simulink model "test_dca"  (R2018a)
settings: Solver=FixedStepAuto  StartTime=0.0  StopTime=4  FixedStep=0.01  RelTol=1e-3
undefined symbols (not defined in the file or in its folder): sigbuilder_block
libraries: qcatlib x2
settings Model: Creator=mengc  LastModifiedBy=mengc

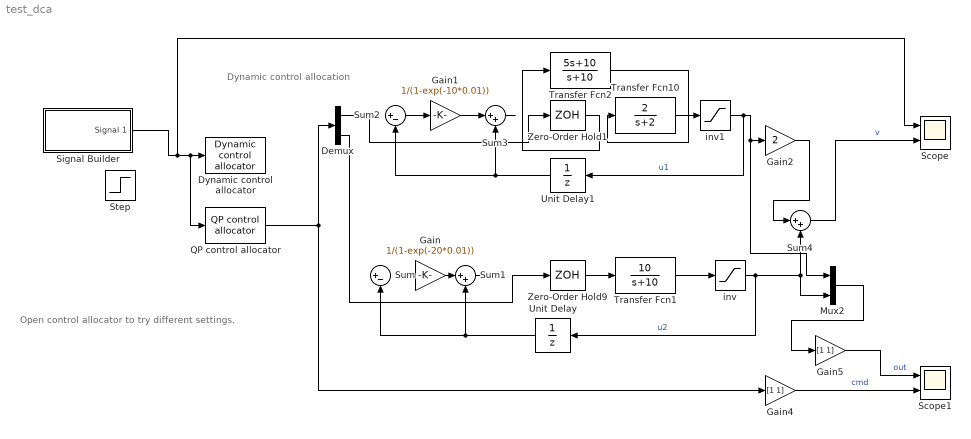
== system test_dca ==
  note: Open control allocator to try different settings.
  note: Dynamic control allocation
  Demux : Demux  Outputs=2
  Dynamic control allocator : qcatlib/Dynamic control allocator  B=[2 1]  plim=[-1 1;-2 2]  rlim=[-1 1;-5 5]  T=0.01  Wv=1  W1=diag([1 1])  W2=diag([8 0])  S=[0 1]'
      settings: SourceProductName=QP Control Allocation Toolbox
  Gain : Gain  Gain=1/(1-exp(-20*0.01))
  Gain1 : Gain  Gain=1/(1-exp(-10*0.01))
  Gain2 : Gain  Gain=2
  Gain4 : Gain  Gain=[1 1]
  Gain5 : Gain  Gain=[1 1]
  Mux2 : Mux  Inputs=2
  QP control allocator : qcatlib/QP control allocator  B=[2 1]  plim=[-1 1;-2 2]  rlim=[-1 1;-5 5]  T=0.01  Wv=1  Wu=diag([1 1])  ud=[0;0]  alg=WLS  imax=100  gam=1e4  tol=1e-4
  Scope : Scope  NumInputPorts=2
  Scope1 : Scope  NumInputPorts=2
  Signal Builder : Subsystem  Tag=STV Subsys  LoadFcn=sigbuilder_block('load',[437.25 153 550.5 358.5 ]);  StartFcn=sigbuilder_block('start');  StopFcn=sigbuilder_block('stop');  ClipboardFcn=sigbuilder_block('clipboard');  mask(Sigbuilder block){tuvar=[0:10]}
      mask help: Simulink:masks:SigbuilderBlock_MD
      mask init:
      | if ~strcmp(get_param(bdroot(gcbh),'SimulationStatus'),'stopped') tuvar = sigbuilder_block('maskInit'); end
      settings: CopyFcn=sigbuilder_block('copy');  DeleteFcn=sigbuilder_block('delete');  ModelCloseFcn=sigbuilder_block('modelClose');  PreSaveFcn=sigbuilder_block('preSave');  PauseFcn=sigbuilder_block('pause');  ContinueFcn=sigbuilder_block('continue');  NameChangeFcn=sigbuilder_block('namechange');  OpenFcn=sigbuilder_block('open',[437.6 199.2 550.4 400 ]);  CloseFcn=sigbuilder_block('close');
      mask Display: plot(0, 0, 100, 100,[2, 2, 32, 32, 2], [68, 8, 8, 68, 68],[32, 2], [38, 38], [32, 19, 2],[53, 60, 44], [32, 17, 17, 2],[16, 16, 31, 31]);txt = getActiveGroup(gcbh);text(2, 100, txt,'verticalAlignment', 'top');
  Step : Step  SampleTime=0.01
  Sum : Sum  Inputs=|+-
  Sum1 : Sum  Inputs=|++
  Sum2 : Sum  Inputs=|+-
  Sum3 : Sum  Inputs=|++
  Sum4 : Sum  Inputs=|++
  Transfer Fcn1 : TransferFcn  Numerator=10  Denominator=[1 10]
  Transfer Fcn10 : TransferFcn  Numerator=2  Denominator=[1 2]
  Transfer Fcn2 : TransferFcn  Numerator=[5 10]  Denominator=[1 10]
  Unit Delay : UnitDelay  SampleTime=-1
  Unit Delay1 : UnitDelay  SampleTime=-1
  Zero-Order Hold1 : ZeroOrderHold  SampleTime=-1
  Zero-Order Hold9 : ZeroOrderHold  SampleTime=-1
  inv : Saturate  UpperLimit=2  LowerLimit=-2
  inv1 : Saturate  UpperLimit=1  LowerLimit=-1
  wires:
  Sum4/1 -> Scope/2  "v"
  Transfer Fcn1/1 -> inv/1
  Sum1/1 -> ?
  Gain/1 -> Sum1/1
  Unit Delay/1 -> Sum/2, Sum1/2
  Demux/2 -> Zero-Order Hold9/1
  inv1/1 -> Mux2/1, Gain2/1, Unit Delay1/1  "u1"
  Transfer Fcn10/1 -> inv1/1
  Sum3/1 -> ?
  Gain1/1 -> Sum3/1
  Unit Delay1/1 -> Sum2/2, Sum3/2
  Demux/1 -> Zero-Order Hold1/1
  Sum2/1 -> Gain1/1
  Zero-Order Hold1/1 -> Transfer Fcn2/1
  inv/1 -> Mux2/2, Sum4/2, Unit Delay/1  "u2"
  Gain2/1 -> Sum4/1
  Gain5/1 -> Scope1/1  "out"
  Gain4/1 -> Scope1/2  "cmd"
  Mux2/1 -> Gain5/1
  Zero-Order Hold9/1 -> Transfer Fcn1/1
  Transfer Fcn2/1 -> Transfer Fcn10/1
  QP control allocator/1 -> Gain4/1, Demux/1
  Signal Builder/1(Signal 1) -> QP control allocator/1, Dynamic control allocator/1, Scope/1

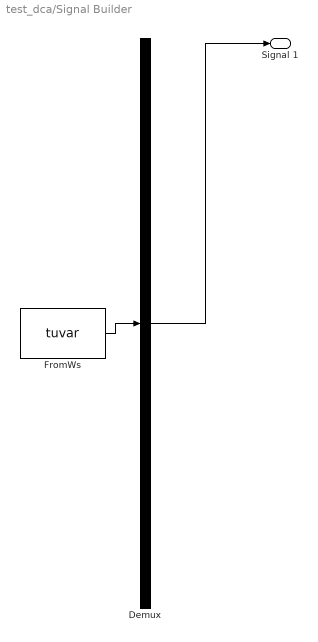
== system test_dca/Signal Builder ==
  Demux : Demux  Tag=STV Demux  Outputs=1
  FromWs : FromWorkspace  Tag=STV FromWs  VariableName=tuvar  SampleTime=0
      SigBuilderData=|
      | common.afterFinalStr = 'Extrapolate'
      | common.sampleTime = 0
      | dataSet.timeRange = [0 10]
      | dataSet.name = 'Group 1'
      | sbobj.Groups.Name = 'Group 1'
      | sbobj.Groups.Signals.Name = 'Signal 1'
      | sbobj.Groups.Signals.XData = [0 1 1.2 6 6 10]
      | sbobj.Groups.Signals.YData = [0 0 1 1 0 0]
  Signal 1 : Outport  Tag=STV Outport
  wires:
  Demux/1 -> Signal 1/1
  FromWs/1 -> Demux/1
